simulink model "SRP"  (R2024b)
settings: Solver=ode5  StartTime=0.0  StopTime=10.0  FixedStep=0.1  RelTol=1e-3
values from neighbouring files (symbols this model uses):
  Ar = [6e-2; 6e-2; 6e-2; 6e-2; 4e-2; 4e-2; 12e-2; 12e-2; 12e-2; 12e-2]    [LabsDCM.m]    (also in Srp_Lab7.m; airdrag.m)
  c = astroConstants(5)    [LabsDCM.m]    (also in Srp_Lab7.m; airdrag.m)
  Ep = deg2rad(epsilon)    [LabsDCM.m]    (also in Srp_Lab7.m = deg2rad(23.45); airdrag.m)
  J = diag([Ix Iy Iz])    [LabsDCM.m]    (also in Srp_Lab7.m; airdrag.m)
  N_B = [ 1,  0,  0 ... (first row only)    [LabsDCM.m]    (also in Srp_Lab7.m; airdrag.m)
  nx = 2*pi()/T    [LabsDCM.m]    (also in Srp_Lab7.m; airdrag.m)
  r_Fi = [ ... (first row only)    [LabsDCM.m]    (also in Srp_Lab7.m; airdrag.m)
  r_sun = astroConstants(2)    [LabsDCM.m]    (also in Srp_Lab7.m; airdrag.m = astroConstants(3))
  rho_d = [0.1; 0.1; 0.1; 0.1; 0.1; 0.1; 0.1; 0.1; 0.1; 0.1]    [LabsDCM.m]    (also in Srp_Lab7.m; airdrag.m)
  rho_s = [0.5; 0.5; 0.5; 0.5; 0.5; 0.5; 0.1; 0.1; 0.1; 0.1]    [LabsDCM.m]    (also in Srp_Lab7.m; airdrag.m)
  W0 = [0.45 0.52 0.55]    [LabsDCM.m]    (also in Srp_Lab7.m; airdrag.m)
libraries: matrix_library x2, vrlib x1
settings Model: Creator=User  LastModifiedBy=User

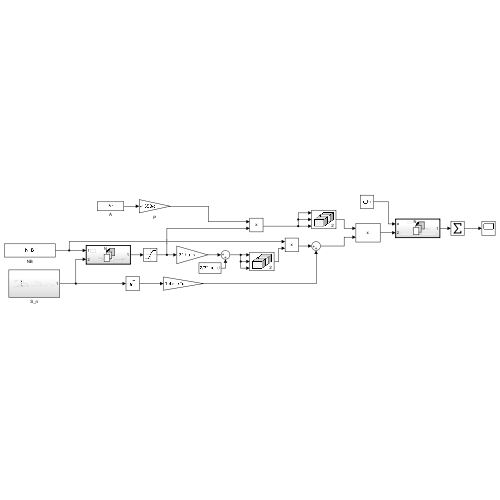
[thumbnail: Simulink's stored preview of the top-level diagram]
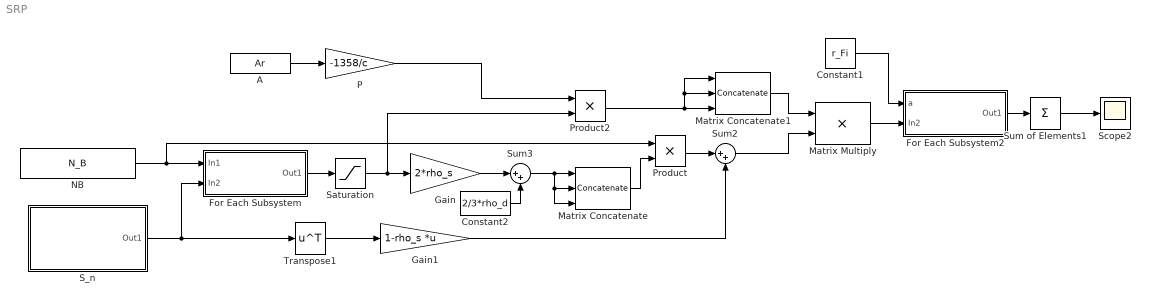
== system SRP ==
  A : Constant  Value=Ar
  Constant1 : Constant  Value=r_Fi
  Constant2 : Constant  Value=2/3*rho_d
  For Each Subsystem : Subsystem  TreatAsAtomicUnit=on
  For Each Subsystem2 : Subsystem  TreatAsAtomicUnit=on
  Gain : Gain  Gain=2*rho_s
  Gain1 : Gain  Gain=1-rho_s  Multiplication=Matrix(K*u)
  Matrix Concatenate : Concatenate  NumInputs=3  Mode=Multidimensional array  ConcatenateDimension=2
  Matrix Concatenate1 : Concatenate  NumInputs=3  Mode=Multidimensional array  ConcatenateDimension=2
  Matrix Multiply : Product
  NB : Constant  Value=N_B
  P : Gain  Gain=-1358/c
  Product : Product
  Product2 : Product
  S_n : Subsystem
  Saturation : Saturate  UpperLimit=inf  LowerLimit=0
  Scope2 : Scope
  Sum of Elements1 : Sum  Inputs=+  CollapseMode=Specified dimension
  Sum2 : Sum  Inputs=|++
  Sum3 : Sum  Inputs=|++
  Transpose1 : Math  Operator=transpose
  wires:
  Gain1/1 -> Sum2/2
  Sum of Elements1/1 -> Scope2/1
  Matrix Concatenate1/1 -> Matrix Multiply/1
  S_n/1(Out1) -> For Each Subsystem/2(In2), Transpose1/1
  Transpose1/1 -> Gain1/1
  A/1 -> P/1
  Constant2/1 -> Sum3/2
  Matrix Multiply/1 -> For Each Subsystem2/2(In2)
  Gain/1 -> Sum3/1
  For Each Subsystem/1(Out1) -> Saturation/1
  Sum3/1 -> Matrix Concatenate/1, Matrix Concatenate/3, Matrix Concatenate/2
  Constant1/1 -> For Each Subsystem2/1(a)
  P/1 -> Product2/1
  Saturation/1 -> Product2/2, Gain/1
  Product2/1 -> Matrix Concatenate1/3, Matrix Concatenate1/2, Matrix Concatenate1/1
  NB/1 -> For Each Subsystem/1(In1), Product/1
  For Each Subsystem2/1(Out1) -> Sum of Elements1/1
  Sum2/1 -> Matrix Multiply/2
  Product/1 -> Sum2/1
  Matrix Concatenate/1 -> Product/2

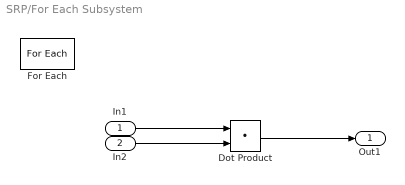
== system SRP/For Each Subsystem ==
  In1 : Inport  Partition=on  PartitionDimension=1  PartitionWidth=1  PartitionOffset=0
  In2 : Inport  Port=2
  Dot Product : DotProduct  OutDataTypeStr=Inherit: Inherit via internal rule
  For Each : ForEach  DisableCoverage=on  SpecifiedNumIters=10
  Out1 : Outport  ConcatenationDimension=1
  wires:
  In1/1 -> Dot Product/1
  Dot Product/1 -> Out1/1
  In2/1 -> Dot Product/2

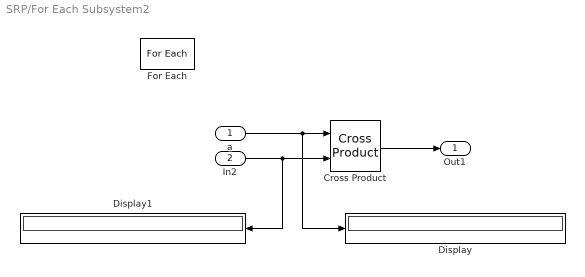
== system SRP/For Each Subsystem2 ==
  a : Inport  Partition=on  PartitionDimension=1  PartitionWidth=1  PartitionOffset=0
  In2 : Inport  Port=2  Partition=on  PartitionDimension=1  PartitionWidth=1  PartitionOffset=0
  Cross Product : matrix_library/Cross Product
  Display : Display
  Display1 : Display
  For Each : ForEach  DisableCoverage=on
  Out1 : Outport  ConcatenationDimension=1
  wires:
  a/1 -> Display/1, Cross Product/1
  In2/1 -> Display1/1, Cross Product/2
  Cross Product/1 -> Out1/1

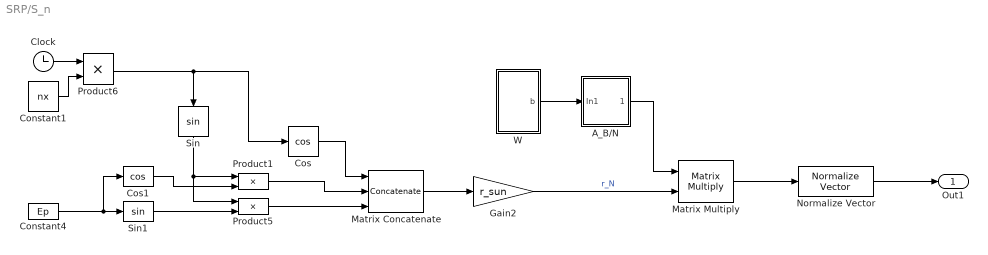
== system SRP/S_n ==
  A_B/N : Subsystem
  Clock : Clock
  Constant1 : Constant  Value=nx
  Constant4 : Constant  Value=Ep
  Cos : Trigonometry  Operator=cos
  Cos1 : Trigonometry  Operator=cos
  Gain2 : Gain  Gain=r_sun
  Matrix Concatenate : Concatenate  NumInputs=3  Mode=Multidimensional array
  Matrix Multiply : Product  Multiplication=Matrix(*)
  Normalize Vector : vrlib/Utilities/Normalize Vector  maxzero=0
  Product1 : Product
  Product5 : Product
  Product6 : Product
  Sin : Trigonometry
  Sin1 : Trigonometry
  W : Subsystem
  Out1 : Outport
  wires:
  A_B/N/1(Out1) -> Matrix Multiply/1
  Constant4/1 -> Cos1/1, Sin1/1
  Sin/1 -> Product5/1, Product1/1
  Product6/1 -> Cos/1, Sin/1
  Gain2/1 -> Matrix Multiply/2  "r_N"
  Cos/1 -> Matrix Concatenate/1
  Cos1/1 -> Product1/2
  W/1(b) -> A_B/N/1(In1)
  Sin1/1 -> Product5/2
  Clock/1 -> Product6/1
  Matrix Concatenate/1 -> Gain2/1
  Constant1/1 -> Product6/2
  Product1/1 -> Matrix Concatenate/2
  Product5/1 -> Matrix Concatenate/3
  Matrix Multiply/1 -> Normalize Vector/1
  Normalize Vector/1 -> Out1/1

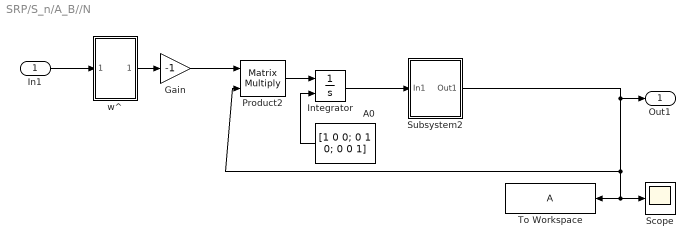
== system SRP/S_n/A_B//N ==
  In1 : Inport
  A0 : Constant  Value=[1 0 0; 0 1 0; 0 0 1]
  Gain : Gain  Gain=-1
  Integrator : Integrator  InitialConditionSource=external
  Product2 : Product  Multiplication=Matrix(*)
  Scope : Scope
  Subsystem2 : Subsystem
  To Workspace : ToWorkspace  VariableName=A  SampleTime=-1
  w^ : Subsystem
  Out1 : Outport
  wires:
  Gain/1 -> Product2/1
  Integrator/1 -> Subsystem2/1(In1)
  Subsystem2/1(Out1) -> To Workspace/1, Scope/1, Product2/2, Out1/1
  In1/1 -> w^/1(In1)
  w^/1(Out1) -> Gain/1
  Product2/1 -> Integrator/1
  A0/1 -> Integrator/2

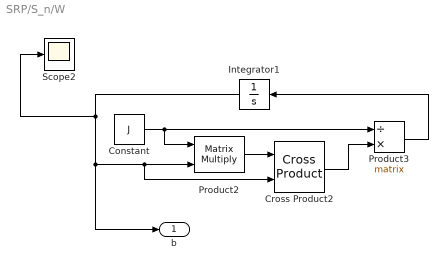
== system SRP/S_n/W ==
  Constant : Constant  Value=J
  Cross Product2 : matrix_library/Cross Product
  Integrator1 : Integrator  InitialCondition=W0
  Product2 : Product  Multiplication=Matrix(*)
  Product3 : Product  Inputs=/*  Multiplication=Matrix(*)
  Scope2 : Scope
  b : Outport
  wires:
  Cross Product2/1 -> Product3/2
  Integrator1/1 -> b/1, Cross Product2/2, Product2/2, Scope2/1
  Constant/1 -> Product2/1, Product3/1
  Product2/1 -> Cross Product2/1
  Product3/1 -> Integrator1/1

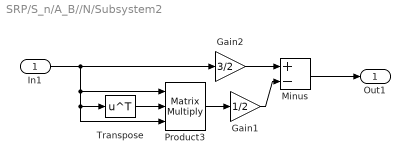
== system SRP/S_n/A_B//N/Subsystem2 ==
  In1 : Inport
  Gain1 : Gain  Gain=1/2
  Gain2 : Gain  Gain=3/2
  Minus : Sum  Inputs=+-
  Product3 : Product  Inputs=3  Multiplication=Matrix(*)
  Transpose : Math  Operator=transpose
  Out1 : Outport
  wires:
  Gain1/1 -> Minus/2
  Gain2/1 -> Minus/1
  In1/1 -> Product3/3, Transpose/1, Product3/1, Gain2/1
  Transpose/1 -> Product3/2
  Product3/1 -> Gain1/1
  Minus/1 -> Out1/1

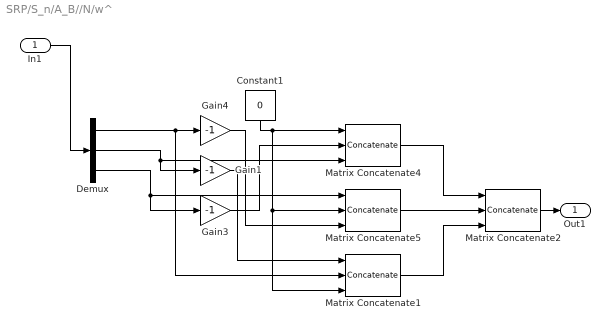
== system SRP/S_n/A_B//N/w^ ==
  In1 : Inport
  Constant1 : Constant  Value=0
  Demux : Demux  Outputs=3
  Gain1 : Gain  Gain=-1
  Gain3 : Gain  Gain=-1
  Gain4 : Gain  Gain=-1
  Matrix Concatenate1 : Concatenate  NumInputs=3  Mode=Multidimensional array  ConcatenateDimension=2
  Matrix Concatenate2 : Concatenate  NumInputs=3  Mode=Multidimensional array
  Matrix Concatenate4 : Concatenate  NumInputs=3  Mode=Multidimensional array  ConcatenateDimension=2
  Matrix Concatenate5 : Concatenate  NumInputs=3  Mode=Multidimensional array  ConcatenateDimension=2
  Out1 : Outport
  wires:
  Matrix Concatenate1/1 -> Matrix Concatenate2/3
  Gain3/1 -> Matrix Concatenate4/2
  Constant1/1 -> Matrix Concatenate4/1, Matrix Concatenate5/2, Matrix Concatenate1/3
  Demux/3 -> Gain3/1, Matrix Concatenate5/1
  Demux/1 -> Gain4/1, Matrix Concatenate1/2
  Matrix Concatenate5/1 -> Matrix Concatenate2/2
  Demux/2 -> Gain1/1, Matrix Concatenate4/3
  Matrix Concatenate4/1 -> Matrix Concatenate2/1
  Gain4/1 -> Matrix Concatenate5/3
  Gain1/1 -> Matrix Concatenate1/1
  Matrix Concatenate2/1 -> Out1/1
  In1/1 -> Demux/1
